simulink model "hard_threshold_fixed_4"  (R2020a)
settings: Solver=VariableStepAuto  StartTime=0.0  StopTime=10  RelTol=1e-3
libraries: simulink x2, dspswit3 x1, hdlsllib x1
settings Model: Creator=sbuccelli  LastModifiedBy=diflo

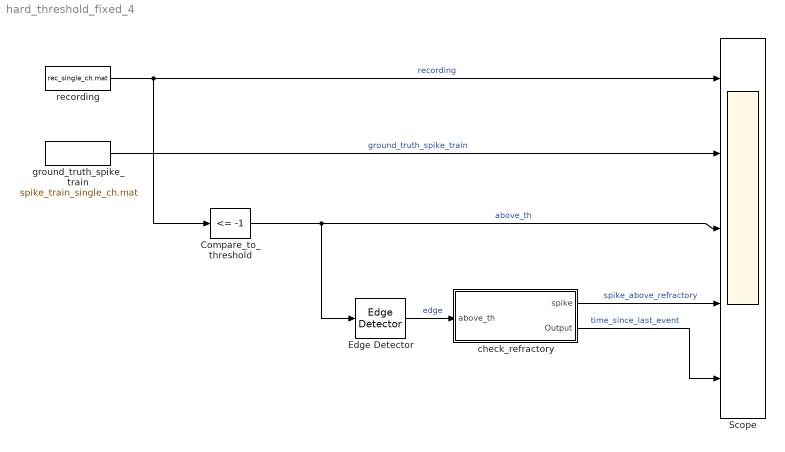
== system hard_threshold_fixed_4 ==
  Compare_to_threshold : simulink/Logic and Bit Operations/Compare To Constant  relop=<=  const=-1  OutDataTypeStr=boolean
  Edge Detector : dspswit3/Edge Detector  InputProcessing=Columns as channels (frame based)
      settings: SourceProductBaseCode=DS
  Scope : Scope  NumInputPorts=5
  check_refractory : Subsystem
  ground_truth_spike_train : FromFile  FileName=spike_train_single_ch.mat  SampleTime=1/32e3
  recording : FromFile  FileName=rec_single_ch.mat  SampleTime=1/32e3
  wires:
  recording/1 -> Compare_to_threshold/1, Scope/1  "recording"
  ground_truth_spike_train/1 -> Scope/2  "ground_truth_spike_train"
  Compare_to_threshold/1 -> Scope/3, Edge Detector/1  "above_th"
  check_refractory/1(spike) -> Scope/4  "spike_above_refractory"
  check_refractory/2(Output) -> Scope/5  "time_since_last_event"
  Edge Detector/1 -> check_refractory/1(above_th)  "edge"

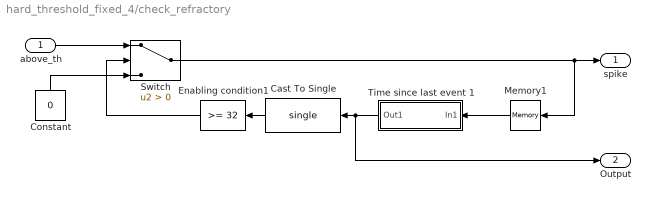
== system hard_threshold_fixed_4/check_refractory ==
  above_th : Inport
  Cast To Single : DataTypeConversion  OutDataTypeStr=single
  Constant : Constant  Value=0
  Enabling condition1 : simulink/Logic and Bit Operations/Compare To Constant  relop=>=  const=32  OutDataTypeStr=boolean
  Memory1 : Memory  InheritSampleTime=on
  Switch : Switch  Criteria=u2 > Threshold
  Time since last event 1 : Subsystem
  spike : Outport
  Output : Outport  Port=2
  wires:
  Switch/1 -> spike/1, Memory1/1
  above_th/1 -> Switch/1
  Memory1/1 -> Time since last event 1/1(In1)
  Time since last event 1/1(Out1) -> Output/1, Cast To Single/1
  Enabling condition1/1 -> Switch/2
  Constant/1 -> Switch/3
  Cast To Single/1 -> Enabling condition1/1

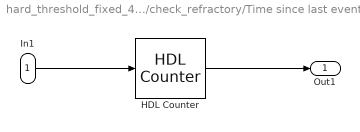
== system hard_threshold_fixed_4/check_refractory/Time since last event 1 ==
  In1 : Inport
  HDL Counter : hdlsllib/Sources/HDL Counter  CountType=Free running  CountInit=1  CountStep=1  CountMax=25  CountFromType=Initial value  CountFrom=1  CountResetPort=on  CountLoadPort=off  CountEnbPort=off  CountDirPort=off  CountDataType=Unsigned  CountWordLen=32  CountFracLen=0  CountSampTime=1
  Out1 : Outport
  wires:
  In1/1 -> HDL Counter/1
  HDL Counter/1 -> Out1/1
